simulink model "ultrasonic"  (R2018b)
settings: Solver=VariableStepAuto  StartTime=0.0  StopTime=10.0  RelTol=1e-3
libraries: simulink x1, arduinolib x1, arduinosensorlib x1
settings Model: Creator=mihii  LastModifiedBy=mihii

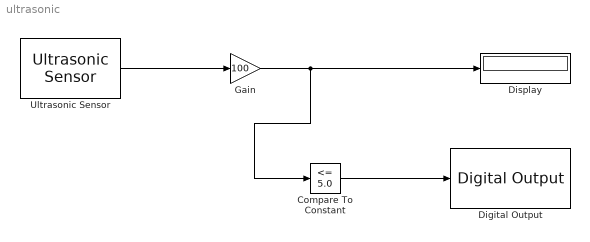
== system ultrasonic ==
  Compare To Constant : simulink/Logic and Bit Operations/Compare To Constant  relop=<=  const=5.0  OutDataTypeStr=boolean
  Digital Output : arduinolib/Digital Output  pinNumber=13  blockPlatform=arduino
  Display : Display
  Gain : Gain  Gain=100
  Ultrasonic Sensor : arduinosensorlib/Ultrasonic Sensor  NumSignalPins=2  TrigPin=4  EchoPin=5  SignalPin=3  SampleTime_=0.1  blockPlatform=ARDUINO
      settings: SourceProductName=Simulink Support Package for Arduino Hardware
  wires:
  Compare To Constant/1 -> Digital Output/1
  Ultrasonic Sensor/1 -> Gain/1
  Gain/1 -> Compare To Constant/1, Display/1
